simulink model "torqueBalancingJointControl"  (Simulink 8.0)
settings: Solver=FixedStepDiscrete  StartTime=0.0  StopTime=CONFIG.SIMULATION_TIME  FixedStep=CONFIG.Ts  RelTol=1e-3
InitFcn:
  | initTorqueBalancing;
undefined symbols (not defined in the file or in its folder): bVectorConstraints, CONFIG, ConstraintsMatrix, DiscIntNeverNeededParam, gain, reg, ROBOT_DOF, sat
libraries: WBToolboxLibrary x45, simulink x2
settings Model: Creator=daniele  LastModifiedBy=gnava
settings DebuggingCC: FcnCallInpInsideContextMsg=EnableAllAsWarning  FrameProcessingCompatibilityMsg=error
settings SFSimCC: SimParseCustomCode=off
settings CodeAppCC: CustomSymbolStrType=$N$R$M_T
settings GRTTargetCC: CodeReplacementLibrary=C89/C90 (ANSI)  CombineOutputUpdateFcns=off  GRTInterface=on

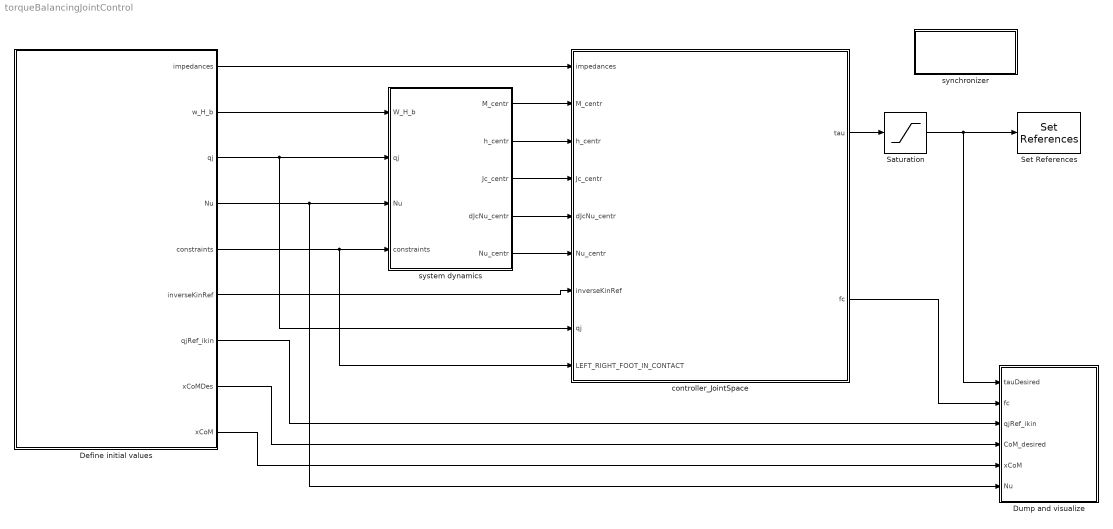
== system torqueBalancingJointControl ==
  Define initial values : Subsystem  Priority=-10
  Dump and visualize : Subsystem
  Saturation : Saturate  UpperLimit=sat.torque  LowerLimit=-sat.torque
  Set References : WBToolboxLibrary/wholeBodyActuators/Set References  controlType=Torque  robotName=WBT_robotName  localName=WBT_modelName  wbiFile=WBT_wbiFilename  wbiList=WBT_wbiList
  controller_JointSpace : Subsystem
  synchronizer : Subsystem
      mask Display: disp('SYNCHRONIZER')
  system dynamics : Subsystem
  wires:
  Define initial values/2(w_H_b) -> system dynamics/1(W_H_b)
  Define initial values/3(qj) -> system dynamics/2(qj), controller_JointSpace/8(qj)
  Define initial values/4(Nu) -> system dynamics/3(Nu), Dump and visualize/6(Nu)
  Define initial values/5(constraints) -> system dynamics/4(constraints), controller_JointSpace/9(LEFT_RIGHT_FOOT_IN_CONTACT)
  system dynamics/1(M_centr) -> controller_JointSpace/2(M_centr)
  system dynamics/2(h_centr) -> controller_JointSpace/3(h_centr)
  system dynamics/3(Jc_centr) -> controller_JointSpace/4(Jc_centr)
  system dynamics/4(dJcNu_centr) -> controller_JointSpace/5(dJcNu_centr)
  system dynamics/5(Nu_centr) -> controller_JointSpace/6(Nu_centr)
  Define initial values/6(inverseKinRef) -> controller_JointSpace/7(inverseKinRef)
  Define initial values/1(impedances) -> controller_JointSpace/1(impedances)
  controller_JointSpace/1("tau ") -> Saturation/1
  Saturation/1 -> Dump and visualize/1(tauDesired), Set References/1
  controller_JointSpace/2(fc) -> Dump and visualize/2(fc)
  Define initial values/7(qjRef_ikin) -> Dump and visualize/3(qjRef_ikin)
  Define initial values/8(xCoMDes) -> Dump and visualize/4(CoM_desired)
  Define initial values/9(xCoM) -> Dump and visualize/5(xCoM)

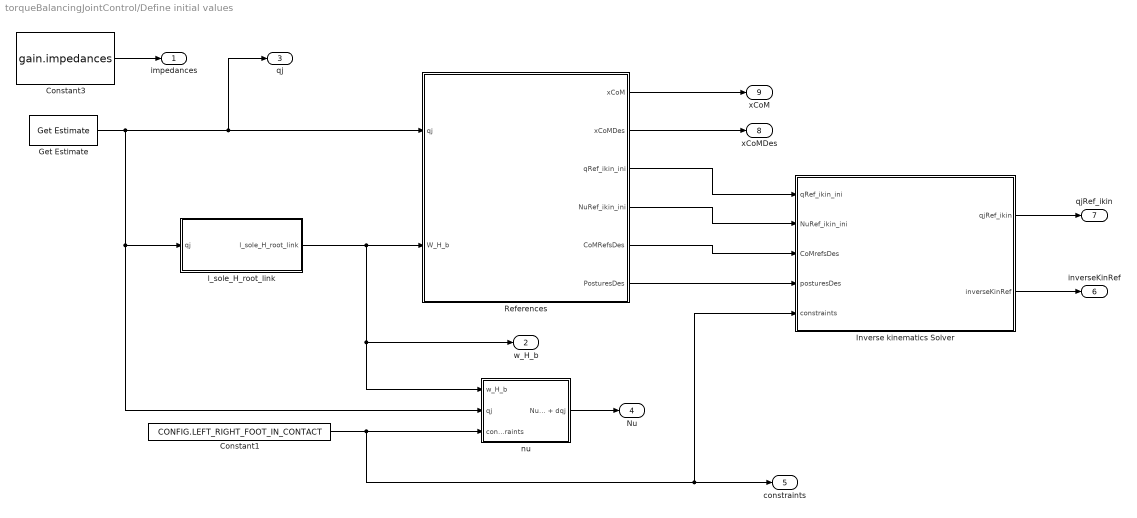
== system torqueBalancingJointControl/Define initial values ==
  Constant1 : Constant  Value=CONFIG.LEFT_RIGHT_FOOT_IN_CONTACT
  Constant3 : Constant  Value=gain.impedances
  Get Estimate : WBToolboxLibrary/wholeBodyStates/Get Estimate  estimateType=Joints Position  robotName=WBT_robotName  localName=WBT_modelName  wbiFile=WBT_wbiFilename  wbiList=WBT_wbiList
  Inverse kinematics Solver : Subsystem
  References : Subsystem
  l_sole_H_root_link : Subsystem
  nu : Subsystem
  impedances : Outport
  w_H_b : Outport  Port=2
  qj : Outport  Port=3
  Nu : Outport  Port=4
  constraints : Outport  Port=5
  inverseKinRef : Outport  Port=6
  qjRef_ikin : Outport  Port=7
  xCoMDes : Outport  Port=8
  xCoM : Outport  Port=9
  wires:
  Constant3/1 -> impedances/1
  Get Estimate/1 -> l_sole_H_root_link/1(qj), nu/2(qj), References/1(qj), qj/1
  l_sole_H_root_link/1(l_sole_H_root_link) -> w_H_b/1, nu/1(w_H_b), References/2(W_H_b)
  nu/1(Nu_b + dqj) -> Nu/1
  References/1(xCoM) -> xCoM/1
  References/2(xCoMDes) -> xCoMDes/1
  Constant1/1 -> Inverse kinematics Solver/5(constraints), constraints/1, nu/3("constraints ")
  Inverse kinematics Solver/1(qjRef_ikin) -> qjRef_ikin/1
  Inverse kinematics Solver/2(inverseKinRef) -> inverseKinRef/1
  References/6(PosturesDes) -> Inverse kinematics Solver/4(posturesDes)
  References/5(CoMRefsDes) -> Inverse kinematics Solver/3(CoMrefsDes)
  References/4(NuRef_ikin_ini) -> Inverse kinematics Solver/2(NuRef_ikin_ini)
  References/3(qRef_ikin_ini) -> Inverse kinematics Solver/1(qRef_ikin_ini)

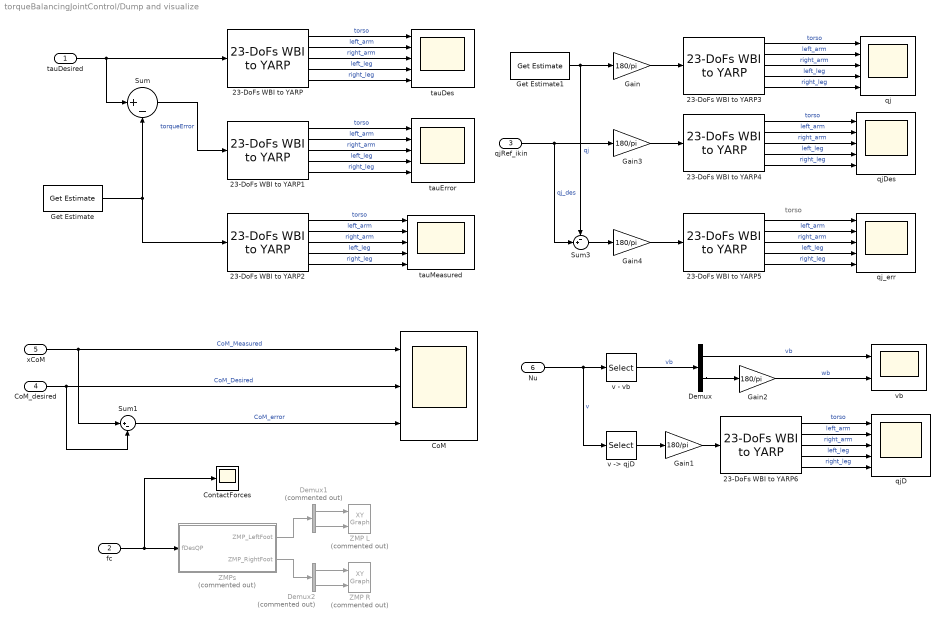
== system torqueBalancingJointControl/Dump and visualize ==
  note: torso
  tauDesired : Inport
  fc : Inport  Port=2
  qjRef_ikin : Inport  Port=3
  CoM_desired : Inport  Port=4
  xCoM : Inport  Port=5
  Nu : Inport  Port=6
  23-DoFs WBI to YARP{,1..6} (7 alike) : WBToolboxLibrary/Utilities/23-DoFs WBI to YARP
  CoM : Scope  NumInputPorts=3
      settings: ShowLegends=on  TimeRange=400  YMin=-0.2~-0.2~-0.045  YMax=0.6~0.6~0.005  SaveName=CoM_data
  ContactForces : Scope
      settings: SaveName=ScopeData2
  Demux : Demux  Outputs=2
  Demux1 : Demux  Commented=on  Outputs=2
  Demux2 : Demux  Commented=on  Outputs=2
  Gain{,1..4} (5 alike) : Gain  Gain=180/pi
  Get Estimate : WBToolboxLibrary/wholeBodyStates/Get Estimate  estimateType=Joints Torque  robotName=WBT_robotName  localName=WBT_modelName  wbiFile=WBT_wbiFilename  wbiList=WBT_wbiList
  Get Estimate1 : WBToolboxLibrary/wholeBodyStates/Get Estimate  estimateType=Joints Position  robotName=WBT_robotName  localName=WBT_modelName  wbiFile=WBT_wbiFilename  wbiList=WBT_wbiList
  Sum : Sum  Inputs=|+-
  Sum1 : Sum  Inputs=|+-
  Sum3 : Sum  Inputs=-+|
  ZMP L : simulink/Sinks/XY Graph  Commented=on  xmin=gain.footSize(1,1)  xmax=gain.footSize(1,2)  ymin=gain.footSize(2,1)  ymax=gain.footSize(2,2)  st=-1
  ZMP R : simulink/Sinks/XY Graph  Commented=on  xmin=gain.footSize(1,1)  xmax=gain.footSize(1,2)  ymin=gain.footSize(2,1)  ymax=gain.footSize(2,2)  st=-1
  ZMPs : Subsystem  Commented=on
  qj : Scope  NumInputPorts=5
      settings: ShowLegends=on  TimeRange=40  YMin=-5~-40~-40~-15~-15  YMax=8~60~60~15~15  SaveName=qj_and_v
  qjD : Scope  NumInputPorts=5
      settings: ShowLegends=on  TimeRange=40  YMin=-1~-0.2~-0.6~-3~-3  YMax=3~0.5~0.3~3~3  SaveName=qj_and_v1
  qjDes : Scope  NumInputPorts=5
      settings: ShowLegends=on  TimeRange=40  YMin=-13.18879~-50.35129~-51.01363~-14.07847~-15.42592  YMax=8.56867~62.73253~62.72359~15.05436~15.88206  SaveName=qj_and_v3
  qj_err : Scope  NumInputPorts=5
      settings: ShowLegends=on  TimeRange=40  YMin=-27.27476~-4.23851~-4.57478~-6.37088~-5.38345  YMax=17.10367~4.06727~2.87419~5.35549~6.40509  SaveName=qj_and_v4
  tauDes : Scope  NumInputPorts=5
      settings: ShowLegends=on  TimeRange=14  YMin=-19.49982~-5.04916~-6.41013~-19.61704~-14.11485  YMax=15.70467~4.10511~5.2534~18.2484~18.38621  SaveName=tauDes
  tauError : Scope  NumInputPorts=5
      settings: ShowLegends=on  TimeRange=90  YMin=-4.41555~-1.22651~-0.86191~-3.55477~-4.30808  YMax=5.88399~0.83922~1.20608~5.47683~6.35708  SaveName=tauError
  tauMeasured : Scope  NumInputPorts=5
      settings: ShowLegends=on  TimeRange=14  YMin=-6~-2.5~-2.5~-6~-6  YMax=5~2~1.5~5~5  SaveName=tauMeasured
  v - vb : Selector  InputPortWidth=ROBOT_DOF+6  IndexOptions=Index vector (dialog)  Indices=[1:6]  OutputSizes=1
  "v -> qjD" : Selector  InputPortWidth=ROBOT_DOF+6  IndexOptions=Index vector (dialog)  Indices=[7:ROBOT_DOF+6]  OutputSizes=1
  vb : Scope  NumInputPorts=2
      settings: ShowLegends=on  TimeRange=40  YMin=-0.02~-1.75  YMax=0.0175~2  SaveName=qj_and_v2
  wires:
  xCoM/1 -> Sum1/1, CoM/1  "CoM_Measured"
  CoM_desired/1 -> Sum1/2, CoM/2  "CoM_Desired"
  Nu/1 -> "v -> qjD"/1, v - vb/1  "v"
  Get Estimate1/1 -> Sum3/1, Gain/1  "qj"
  Gain/1 -> 23-DoFs WBI to YARP3/1
  23-DoFs WBI to YARP3/5 -> qj/5  "right_leg"
  23-DoFs WBI to YARP3/1 -> qj/1  "torso"
  23-DoFs WBI to YARP3/2 -> qj/2  "left_arm"
  23-DoFs WBI to YARP3/4 -> qj/4  "left_leg"
  23-DoFs WBI to YARP3/3 -> qj/3  "right_arm"
  23-DoFs WBI to YARP6/5 -> qjD/5  "right_leg"
  23-DoFs WBI to YARP6/1 -> qjD/1  "torso"
  23-DoFs WBI to YARP6/2 -> qjD/2  "left_arm"
  23-DoFs WBI to YARP6/4 -> qjD/4  "left_leg"
  23-DoFs WBI to YARP6/3 -> qjD/3  "right_arm"
  "v -> qjD"/1 -> Gain1/1
  v - vb/1 -> Demux/1  "vb"
  Demux/1 -> vb/1  "vb"
  Demux/2 -> Gain2/1
  Gain1/1 -> 23-DoFs WBI to YARP6/1
  Gain2/1 -> vb/2  "wb"
  fc/1 -> ContactForces/1, ZMPs/1(fDesQP)
  ZMPs/1(ZMP_LeftFoot) -> Demux1/1
  ZMPs/2(ZMP_RightFoot) -> Demux2/1
  Demux1/1 -> ZMP L/1
  Demux1/2 -> ZMP L/2
  Demux2/1 -> ZMP R/1
  Demux2/2 -> ZMP R/2
  tauDesired/1 -> Sum/1, 23-DoFs WBI to YARP/1
  Get Estimate/1 -> 23-DoFs WBI to YARP2/1, Sum/2
  23-DoFs WBI to YARP/5 -> tauDes/5  "right_leg"
  23-DoFs WBI to YARP/1 -> tauDes/1  "torso"
  23-DoFs WBI to YARP/2 -> tauDes/2  "left_arm"
  23-DoFs WBI to YARP/4 -> tauDes/4  "left_leg"
  23-DoFs WBI to YARP/3 -> tauDes/3  "right_arm"
  23-DoFs WBI to YARP1/5 -> tauError/5  "right_leg"
  23-DoFs WBI to YARP1/1 -> tauError/1  "torso"
  23-DoFs WBI to YARP1/2 -> tauError/2  "left_arm"
  23-DoFs WBI to YARP1/4 -> tauError/4  "left_leg"
  23-DoFs WBI to YARP1/3 -> tauError/3  "right_arm"
  Sum/1 -> 23-DoFs WBI to YARP1/1  "torqueError"
  23-DoFs WBI to YARP2/5 -> tauMeasured/5  "right_leg"
  23-DoFs WBI to YARP2/1 -> tauMeasured/1  "torso"
  23-DoFs WBI to YARP2/2 -> tauMeasured/2  "left_arm"
  23-DoFs WBI to YARP2/4 -> tauMeasured/4  "left_leg"
  23-DoFs WBI to YARP2/3 -> tauMeasured/3  "right_arm"
  23-DoFs WBI to YARP4/5 -> qjDes/5  "right_leg"
  23-DoFs WBI to YARP4/1 -> qjDes/1  "torso"
  23-DoFs WBI to YARP4/2 -> qjDes/2  "left_arm"
  23-DoFs WBI to YARP4/4 -> qjDes/4  "left_leg"
  23-DoFs WBI to YARP4/3 -> qjDes/3  "right_arm"
  Gain4/1 -> 23-DoFs WBI to YARP5/1
  23-DoFs WBI to YARP5/5 -> qj_err/5  "right_leg"
  23-DoFs WBI to YARP5/2 -> qj_err/2  "left_arm"
  23-DoFs WBI to YARP5/4 -> qj_err/4  "left_leg"
  23-DoFs WBI to YARP5/3 -> qj_err/3  "right_arm"
  Sum3/1 -> Gain4/1
  qjRef_ikin/1 -> Gain3/1, Sum3/2  "qj_des"
  Gain3/1 -> 23-DoFs WBI to YARP4/1
  23-DoFs WBI to YARP5/1 -> qj_err/1
  Sum1/1 -> CoM/3  "CoM_error"

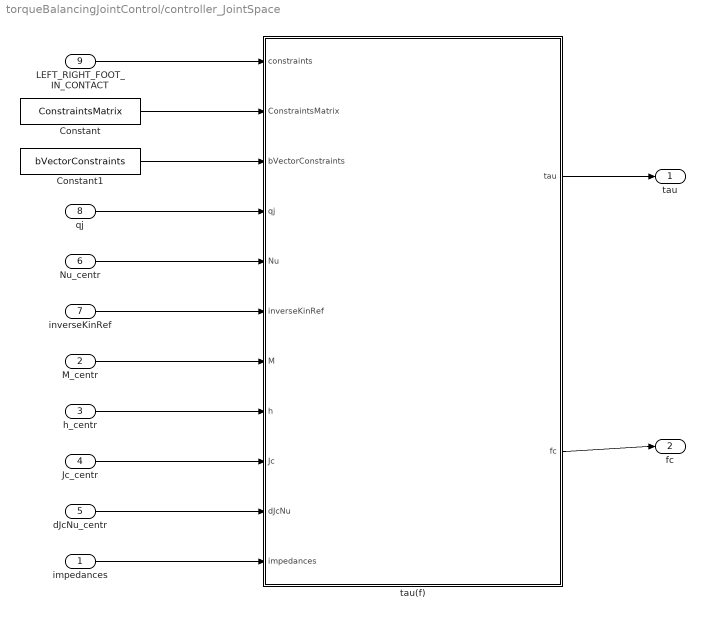
== system torqueBalancingJointControl/controller_JointSpace ==
  impedances : Inport
  M_centr : Inport  Port=2
  h_centr : Inport  Port=3
  Jc_centr : Inport  Port=4
  dJcNu_centr : Inport  Port=5
  Nu_centr : Inport  Port=6
  inverseKinRef : Inport  Port=7
  qj : Inport  Port=8
  LEFT_RIGHT_FOOT_IN_CONTACT : Inport  Port=9
  Constant : Constant  Value=ConstraintsMatrix
  Constant1 : Constant  Value=bVectorConstraints
  "tau(f) " : MATLAB Function  TreatAsAtomicUnit=on
  "tau " : Outport
  fc : Outport  Port=2
  wires:
  LEFT_RIGHT_FOOT_IN_CONTACT/1 -> "tau(f) "/1(constraints)
  M_centr/1 -> "tau(f) "/7(M)
  h_centr/1 -> "tau(f) "/8(h)
  Constant/1 -> "tau(f) "/2(ConstraintsMatrix)
  Constant1/1 -> "tau(f) "/3(bVectorConstraints)
  Jc_centr/1 -> "tau(f) "/9(Jc)
  dJcNu_centr/1 -> "tau(f) "/10(dJcNu)
  Nu_centr/1 -> "tau(f) "/5(Nu)
  impedances/1 -> "tau(f) "/11(impedances)
  "tau(f) "/1(tau) -> "tau "/1
  qj/1 -> "tau(f) "/4(qj)
  inverseKinRef/1 -> "tau(f) "/6(inverseKinRef)
  "tau(f) "/2(fc) -> fc/1

== system torqueBalancingJointControl/synchronizer ==
  Real Time Synchronizer : WBToolboxLibrary/Utilities/Real Time Synchronizer  Commented=on  period=CONFIG.Ts
  Simulator Synchronizer : WBToolboxLibrary/Utilities/Simulator Synchronizer  period=CONFIG.Ts  serverPortName='/clock/rpc'  clientPortName='/WBT_synchronizer/rpc:o'

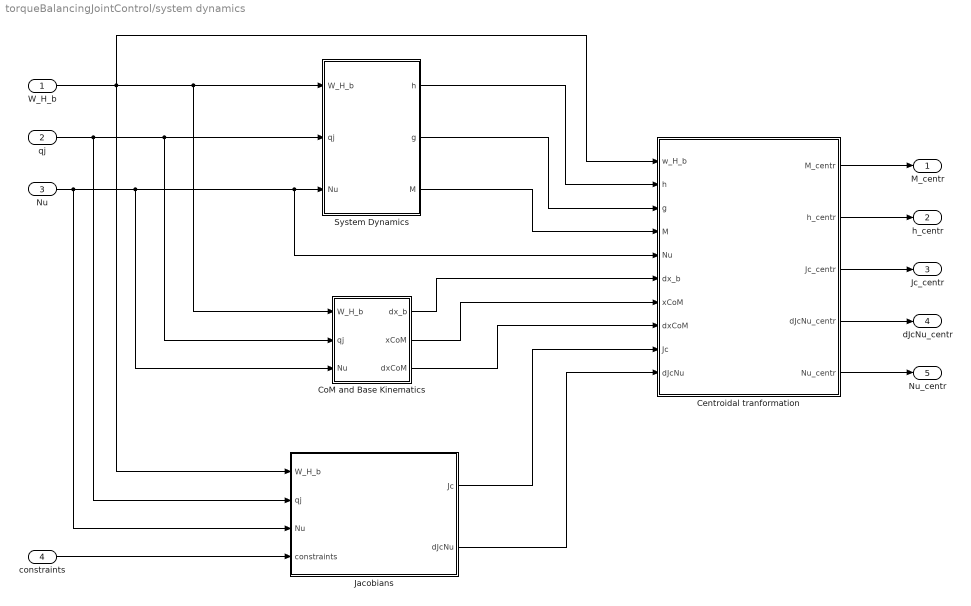
== system torqueBalancingJointControl/system dynamics ==
  W_H_b : Inport
  qj : Inport  Port=2
  Nu : Inport  Port=3
  constraints : Inport  Port=4
  Centroidal tranformation : Subsystem
  CoM and Base Kinematics : Subsystem
  Jacobians : Subsystem
  System Dynamics : Subsystem
  M_centr : Outport
  h_centr : Outport  Port=2
  Jc_centr : Outport  Port=3
  dJcNu_centr : Outport  Port=4
  Nu_centr : Outport  Port=5
  wires:
  Jacobians/2(dJcNu) -> Centroidal tranformation/10(dJcNu)
  Centroidal tranformation/1(M_centr) -> M_centr/1
  System Dynamics/1(h) -> Centroidal tranformation/2(h)
  System Dynamics/2(g) -> Centroidal tranformation/3(g)
  System Dynamics/3(M) -> Centroidal tranformation/4(M)
  CoM and Base Kinematics/1(dx_b) -> Centroidal tranformation/6(dx_b)
  CoM and Base Kinematics/2(xCoM) -> Centroidal tranformation/7(xCoM)
  CoM and Base Kinematics/3(dxCoM) -> Centroidal tranformation/8(dxCoM)
  Jacobians/1(Jc) -> Centroidal tranformation/9(Jc)
  qj/1 -> Jacobians/2(qj), CoM and Base Kinematics/2(qj), System Dynamics/2(qj)
  Nu/1 -> Jacobians/3(Nu), CoM and Base Kinematics/3(Nu), Centroidal tranformation/5(Nu), System Dynamics/3(Nu)
  W_H_b/1 -> Centroidal tranformation/1(w_H_b), Jacobians/1(W_H_b), System Dynamics/1(W_H_b), CoM and Base Kinematics/1(W_H_b)
  Centroidal tranformation/3(Jc_centr) -> Jc_centr/1
  Centroidal tranformation/2(h_centr) -> h_centr/1
  constraints/1 -> Jacobians/4(constraints)
  Centroidal tranformation/5(Nu_centr) -> Nu_centr/1
  Centroidal tranformation/4(dJcNu_centr) -> dJcNu_centr/1

== system torqueBalancingJointControl/Define initial values/Inverse kinematics Solver ==
  qRef_ikin_ini : Inport
  NuRef_ikin_ini : Inport  Port=2
  CoMrefsDes : Inport  Port=3
  posturesDes : Inport  Port=4
  constraints : Inport  Port=5
  Generate ikin Errors : Subsystem
  ikin visualizer : Subsystem
  ikin_DoubleIntegrator : Subsystem
  ikin_utilities : Subsystem
  trajectoryGeneratorCoM : MATLAB Function  TreatAsAtomicUnit=on
  qjRef_ikin : Outport
  inverseKinRef : Outport  Port=2
  wires:
  Generate ikin Errors/1(iKinFeetCorr) -> trajectoryGeneratorCoM/1(iKinFeetCorr), ikin visualizer/1(Ikin_feetCorr)
  Generate ikin Errors/2(iKinComCorr) -> trajectoryGeneratorCoM/2(iKinComCorr), ikin visualizer/2(Ikin_CoMCorr)
  Generate ikin Errors/3(iKinPostCorr) -> ikin visualizer/3(Ikin_PostCorr), trajectoryGeneratorCoM/3(iKinPostCorr)
  ikin_DoubleIntegrator/2(qRef_ikin) -> ikin_utilities/1(qRef_ikin), Generate ikin Errors/12(qRef_ikin)
  ikin_DoubleIntegrator/1(NuRef_ikin) -> ikin_utilities/2(NuRef_ikin), Generate ikin Errors/11(NuRef_iKin)
  qRef_ikin_ini/1 -> ikin_DoubleIntegrator/3(qRef_ikin_init), ikin_utilities/3(qRef_ikin_init)
  CoMrefsDes/1 -> Generate ikin Errors/1(CoMrefsDes)
  posturesDes/1 -> Generate ikin Errors/2(posturesDes)
  ikin_utilities/1(Jlsole) -> Generate ikin Errors/3(Jlfoot), trajectoryGeneratorCoM/4(J_lfoot)
  ikin_utilities/2(Jrsole) -> trajectoryGeneratorCoM/5(J_rfoot), Generate ikin Errors/4(Jrfoot)
  ikin_utilities/3(JCoM) -> Generate ikin Errors/5(JCoM), trajectoryGeneratorCoM/6(J_com)
  ikin_utilities/4(deltaRFootPos) -> Generate ikin Errors/6(rfootPos)
  ikin_utilities/5(deltaLFootPos) -> Generate ikin Errors/7(lfootPos)
  ikin_utilities/6(CoMPos) -> Generate ikin Errors/8(CoMPos)
  ikin_utilities/7(deltaLFootOri) -> Generate ikin Errors/9(lfootOri)
  ikin_utilities/8(deltaRFootOri) -> Generate ikin Errors/10(rfootOri)
  NuRef_ikin_ini/1 -> ikin_DoubleIntegrator/2(Nu_ikin_init)
  trajectoryGeneratorCoM/1(dNuRef_ikin) -> ikin_DoubleIntegrator/1(dNuRef_ikin)
  constraints/1 -> trajectoryGeneratorCoM/10(constraints)
  ikin_utilities/9(dJlfootNu) -> trajectoryGeneratorCoM/7(dJcNu_lf)
  ikin_utilities/10(dJrfootNu) -> trajectoryGeneratorCoM/8(dJcNu_rf)
  ikin_utilities/11(dJCoMNu) -> trajectoryGeneratorCoM/9(dJ_comNu)
  ikin_DoubleIntegrator/3(inverseKinRef) -> inverseKinRef/1
  ikin_DoubleIntegrator/4(qjRef_ikin) -> qjRef_ikin/1

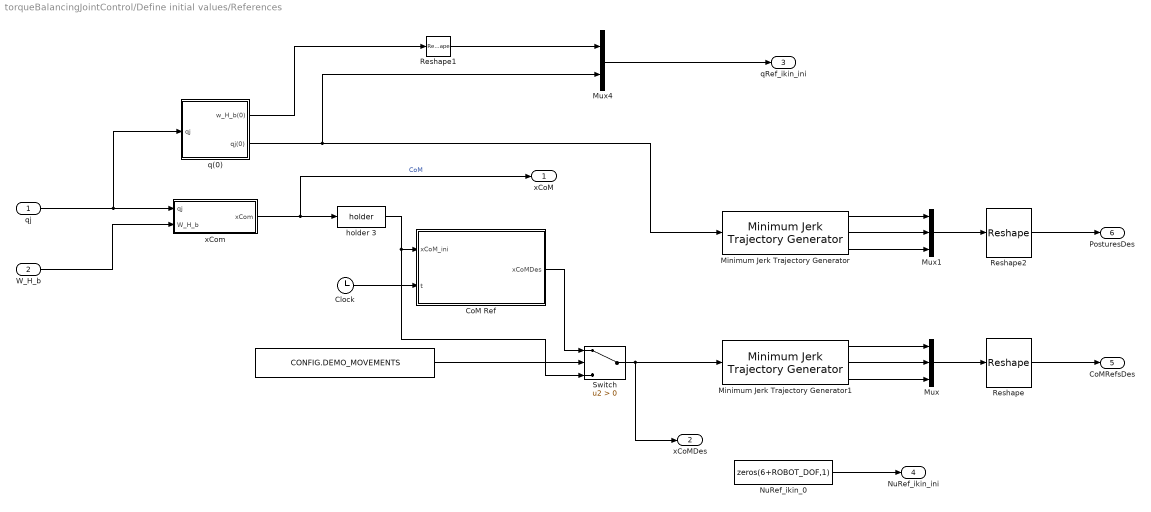
== system torqueBalancingJointControl/Define initial values/References ==
  qj : Inport
  W_H_b : Inport  Port=2
  " " : Constant  Value=CONFIG.DEMO_MOVEMENTS
  Clock : Clock
  CoM Ref : MATLAB Function  TreatAsAtomicUnit=on
  Minimum Jerk Trajectory Generator : WBToolboxLibrary/Utilities/Minimum Jerk Trajectory Generator  externalSettlingTime=off  settlingTime=3  sampleTime=CONFIG.Ts  firstDerivatives=on  secondDerivatives=on  explicitInitialValue=off
  Minimum Jerk Trajectory Generator1 : WBToolboxLibrary/Utilities/Minimum Jerk Trajectory Generator  externalSettlingTime=off  settlingTime=3  sampleTime=CONFIG.Ts  firstDerivatives=on  secondDerivatives=on  explicitInitialValue=off
  Mux : Mux  Inputs=3
  Mux1 : Mux  Inputs=3
  Mux4 : Mux  Inputs=2
  NuRef_ikin_0 : Constant  Value=zeros(6+ROBOT_DOF,1)
  Reshape : Reshape  OutputDimensionality=Customize  OutputDimensions=[3,3]
  Reshape1 : Reshape
  Reshape2 : Reshape  OutputDimensionality=Customize  OutputDimensions=[ROBOT_DOF,3]
  Switch : Switch  Criteria=u2 > Threshold
  holder 3 : WBToolboxLibrary/Utilities/holder 
  q(0) : Subsystem
  xCom : Subsystem  Priority=-2
  xCoM : Outport
  xCoMDes : Outport  Port=2
  qRef_ikin_ini : Outport  Port=3
  NuRef_ikin_ini : Outport  Port=4
  CoMRefsDes : Outport  Port=5
  PosturesDes : Outport  Port=6
  wires:
  xCom/1(xCom) -> xCoM/1, holder 3/1  "CoM"
  qj/1 -> xCom/1(qj), q(0)/1(qj)
  Reshape1/1 -> Mux4/1
  q(0)/1(w_H_b(0)) -> Reshape1/1
  q(0)/2(qj(0)) -> Minimum Jerk Trajectory Generator/1, Mux4/2
  Mux4/1 -> qRef_ikin_ini/1
  Minimum Jerk Trajectory Generator1/1 -> Mux/1
  Minimum Jerk Trajectory Generator1/2 -> Mux/2
  Minimum Jerk Trajectory Generator1/3 -> Mux/3
  Mux/1 -> Reshape/1
  Minimum Jerk Trajectory Generator/1 -> Mux1/1
  Minimum Jerk Trajectory Generator/2 -> Mux1/2
  Minimum Jerk Trajectory Generator/3 -> Mux1/3
  Mux1/1 -> Reshape2/1
  NuRef_ikin_0/1 -> NuRef_ikin_ini/1
  Reshape2/1 -> PosturesDes/1
  Reshape/1 -> CoMRefsDes/1
  W_H_b/1 -> xCom/2(W_H_b)
  " "/1 -> Switch/2
  holder 3/1 -> Switch/3, CoM Ref/1(xCoM_ini)
  Switch/1 -> xCoMDes/1, Minimum Jerk Trajectory Generator1/1
  Clock/1 -> CoM Ref/2(t)
  CoM Ref/1(xCoMDes) -> Switch/1

== system torqueBalancingJointControl/Define initial values/l_sole_H_root_link ==
  qj : Inport
  Constant5 : Constant  Value=eye(4)
  Constant6 : Constant  Value=eye(4)
  Inv\* : Product  Inputs=/*  Multiplication=Matrix(*)
  l_sole : WBToolboxLibrary/wholeBodyModel/Kinematics/Forward Kinematics  frameName='l_sole'  robotName=WBT_robotName  localName=WBT_modelName  wbiFile=WBT_wbiFilename  wbiList=WBT_wbiList
  root_link : WBToolboxLibrary/wholeBodyModel/Kinematics/Forward Kinematics  frameName='root_link'  robotName=WBT_robotName  localName=WBT_modelName  wbiFile=WBT_wbiFilename  wbiList=WBT_wbiList
  l_sole_H_root_link : Outport
  wires:
  Constant5/1 -> l_sole/1
  Inv\*/1 -> l_sole_H_root_link/1  "l_sole_H_root_link"
  l_sole/1 -> Inv\*/1
  Constant6/1 -> root_link/1
  qj/1 -> root_link/2, l_sole/2
  root_link/1 -> Inv\*/2

== system torqueBalancingJointControl/Define initial values/nu ==
  w_H_b : Inport
  qj : Inport  Port=2
  "constraints " : Inport  Port=3
  Get Estimate : WBToolboxLibrary/wholeBodyStates/Get Estimate  estimateType=Joints Velocity  robotName=WBT_robotName  localName=WBT_modelName  wbiFile=WBT_wbiFilename  wbiList=WBT_wbiList
  Jacobian l_sole : WBToolboxLibrary/wholeBodyModel/Jacobians/Jacobian  frameName='l_sole'  robotName=WBT_robotName  localName=WBT_modelName  wbiFile=WBT_wbiFilename  wbiList=WBT_wbiList
  Jacobian r_sole : WBToolboxLibrary/wholeBodyModel/Jacobians/Jacobian  frameName='r_sole'  robotName=WBT_robotName  localName=WBT_modelName  wbiFile=WBT_wbiFilename  wbiList=WBT_wbiList
  Mux : Mux  Inputs=2
  genBaseVelocity : MATLAB Function  TreatAsAtomicUnit=on
  Nu_b + dqj : Outport
  wires:
  Get Estimate/1 -> genBaseVelocity/4(dq), Mux/2
  Mux/1 -> Nu_b + dqj/1
  Jacobian r_sole/1 -> genBaseVelocity/2(JcRightFoot)
  "constraints "/1 -> genBaseVelocity/3(Constraints)
  genBaseVelocity/1(Nu_base) -> Mux/1
  Jacobian l_sole/1 -> genBaseVelocity/1(JcLeftFoot)
  qj/1 -> Jacobian l_sole/2, Jacobian r_sole/2
  w_H_b/1 -> Jacobian r_sole/1, Jacobian l_sole/1

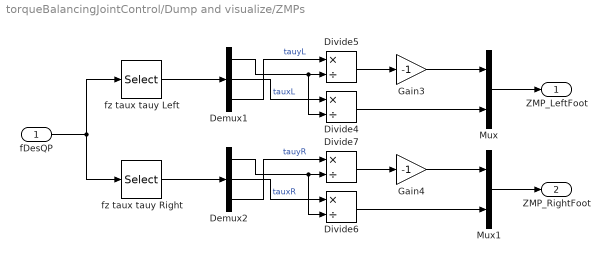
== system torqueBalancingJointControl/Dump and visualize/ZMPs ==
  fDesQP : Inport
  Demux1 : Demux  Outputs=3
  Demux2 : Demux  Outputs=3
  Divide{4..7} (4 alike) : Product  Inputs=*/
  Gain3 : Gain  Gain=-1
  Gain4 : Gain  Gain=-1
  Mux : Mux  Inputs=2
  Mux1 : Mux  Inputs=2
  fz taux tauy Left : Selector  InputPortWidth=12  IndexOptions=Index vector (dialog)  Indices=[3 4 5]  OutputSizes=1
  fz taux tauy Right : Selector  InputPortWidth=12  IndexOptions=Index vector (dialog)  Indices=[9 10 11]  OutputSizes=1
  ZMP_LeftFoot : Outport
  ZMP_RightFoot : Outport  Port=2
  wires:
  fz taux tauy Left/1 -> Demux1/1
  Demux1/1 -> Divide4/2, Divide5/2
  Divide7/1 -> Gain4/1
  Divide4/1 -> Mux/2
  Divide5/1 -> Gain3/1
  fz taux tauy Right/1 -> Demux2/1
  Demux2/1 -> Divide6/2, Divide7/2
  fDesQP/1 -> fz taux tauy Left/1, fz taux tauy Right/1
  Gain3/1 -> Mux/1
  Mux/1 -> ZMP_LeftFoot/1
  Divide6/1 -> Mux1/2
  Gain4/1 -> Mux1/1
  Mux1/1 -> ZMP_RightFoot/1
  Demux1/2 -> Divide4/1  "tauxL"
  Demux1/3 -> Divide5/1  "tauyL"
  Demux2/2 -> Divide6/1  "tauxR"
  Demux2/3 -> Divide7/1  "tauyR"

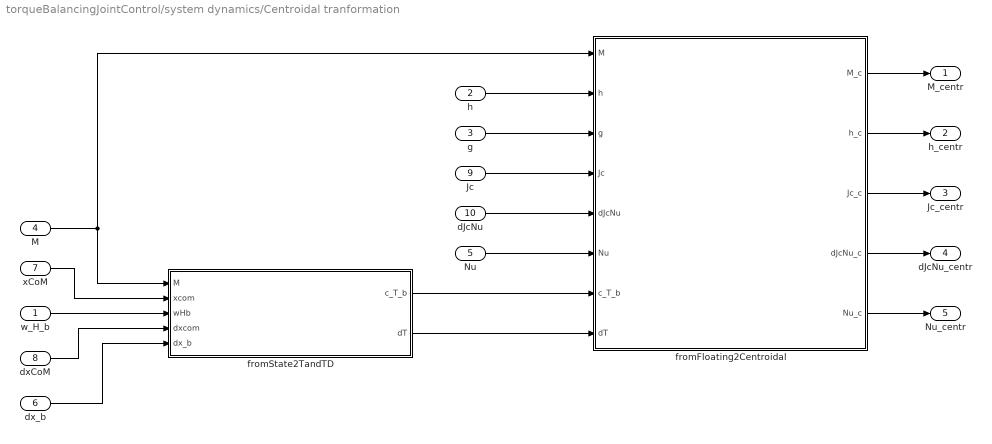
== system torqueBalancingJointControl/system dynamics/Centroidal tranformation ==
  w_H_b : Inport
  h : Inport  Port=2
  g : Inport  Port=3
  M : Inport  Port=4
  Nu : Inport  Port=5
  dx_b : Inport  Port=6
  xCoM : Inport  Port=7
  dxCoM : Inport  Port=8
  Jc : Inport  Port=9
  dJcNu : Inport  Port=10
  fromFloating2Centroidal : MATLAB Function  TreatAsAtomicUnit=on
  fromState2TandTD : MATLAB Function  TreatAsAtomicUnit=on
  M_centr : Outport
  h_centr : Outport  Port=2
  Jc_centr : Outport  Port=3
  dJcNu_centr : Outport  Port=4
  Nu_centr : Outport  Port=5
  wires:
  Nu/1 -> fromFloating2Centroidal/6(Nu)
  dx_b/1 -> fromState2TandTD/5(dx_b)
  xCoM/1 -> fromState2TandTD/2(xcom)
  fromState2TandTD/2(dT) -> fromFloating2Centroidal/8(dT)
  h/1 -> fromFloating2Centroidal/2(h)
  g/1 -> fromFloating2Centroidal/3(g)
  dxCoM/1 -> fromState2TandTD/4(dxcom)
  w_H_b/1 -> fromState2TandTD/3(wHb)
  fromState2TandTD/1(c_T_b) -> fromFloating2Centroidal/7(c_T_b)
  dJcNu/1 -> fromFloating2Centroidal/5(dJcNu)
  Jc/1 -> fromFloating2Centroidal/4(Jc)
  M/1 -> fromState2TandTD/1(M), fromFloating2Centroidal/1(M)
  fromFloating2Centroidal/1(M_c) -> M_centr/1
  fromFloating2Centroidal/2(h_c) -> h_centr/1
  fromFloating2Centroidal/3(Jc_c) -> Jc_centr/1
  fromFloating2Centroidal/4(dJcNu_c) -> dJcNu_centr/1
  fromFloating2Centroidal/5(Nu_c) -> Nu_centr/1

== system torqueBalancingJointControl/system dynamics/CoM and Base Kinematics ==
  W_H_b : Inport
  qj : Inport  Port=2
  Nu : Inport  Port=3
  "CoM6D ->  CoMXYZ1" : Selector  InputPortWidth=6  IndexOptions=Index vector (dialog)  Indices=[1 2 3]  OutputSizes=1
  "CoM6D ->  CoMXYZ4" : Selector  InputPortWidth=6+ROBOT_DOF  IndexOptions=Index vector (dialog)  Indices=[1 2 3]  OutputSizes=1
  "CoM6D ->  CoMXYZ5" : Selector  NumberOfDimensions=2  InputPortWidth=7  IndexOptions=Index vector (dialog),Index vector (dialog)  Indices=[1 2 3],[4]  OutputSizes=1,1
  Jacobian CoM : WBToolboxLibrary/wholeBodyModel/Jacobians/Jacobian  frameName='com'  robotName=WBT_robotName  localName=WBT_modelName  wbiFile=WBT_wbiFilename  wbiList=WBT_wbiList
  JcNu : Product  Multiplication=Matrix(*)
  com : WBToolboxLibrary/wholeBodyModel/Kinematics/Forward Kinematics  frameName='com'  robotName=WBT_robotName  localName=WBT_modelName  wbiFile=WBT_wbiFilename  wbiList=WBT_wbiList
  dx_b : Outport
  xCoM : Outport  Port=2
  dxCoM : Outport  Port=3
  wires:
  qj/1 -> Jacobian CoM/2, com/2
  "CoM6D ->  CoMXYZ4"/1 -> dx_b/1
  com/1 -> "CoM6D ->  CoMXYZ5"/1
  "CoM6D ->  CoMXYZ5"/1 -> xCoM/1
  Jacobian CoM/1 -> JcNu/1
  Nu/1 -> JcNu/2, "CoM6D ->  CoMXYZ4"/1
  W_H_b/1 -> Jacobian CoM/1, com/1
  JcNu/1 -> "CoM6D ->  CoMXYZ1"/1
  "CoM6D ->  CoMXYZ1"/1 -> dxCoM/1

== system torqueBalancingJointControl/system dynamics/Jacobians ==
  W_H_b : Inport
  qj : Inport  Port=2
  Nu : Inport  Port=3
  constraints : Inport  Port=4
  "CoM6D ->  CoMXYZ3" : Selector  InputPortWidth=6+ROBOT_DOF  IndexOptions=Index vector (dialog)  Indices=[7:6+ROBOT_DOF]  OutputSizes=1
  "CoM6D ->  CoMXYZ4" : Selector  InputPortWidth=6+ROBOT_DOF  IndexOptions=Index vector (dialog)  Indices=[1 2 3 4 5 6]  OutputSizes=1
  DotJ Nu lFoot : WBToolboxLibrary/wholeBodyModel/Jacobians/DotJ Nu  frameName='l_sole'  robotName=WBT_robotName  localName=WBT_modelName  wbiFile=WBT_wbiFilename  wbiList=WBT_wbiList
  DotJ Nu rFoot : WBToolboxLibrary/wholeBodyModel/Jacobians/DotJ Nu  frameName='r_sole'  robotName=WBT_robotName  localName=WBT_modelName  wbiFile=WBT_wbiFilename  wbiList=WBT_wbiList
  Jacobian lFoot : WBToolboxLibrary/wholeBodyModel/Jacobians/Jacobian  frameName='l_sole'  robotName=WBT_robotName  localName=WBT_modelName  wbiFile=WBT_wbiFilename  wbiList=WBT_wbiList
  Jacobian rFoot : WBToolboxLibrary/wholeBodyModel/Jacobians/Jacobian  frameName='r_sole'  robotName=WBT_robotName  localName=WBT_modelName  wbiFile=WBT_wbiFilename  wbiList=WBT_wbiList
  composingSmoothJacobians : MATLAB Function  TreatAsAtomicUnit=on
  Jc : Outport
  dJcNu : Outport  Port=2
  wires:
  composingSmoothJacobians/1(Jc) -> Jc/1
  W_H_b/1 -> DotJ Nu rFoot/1, DotJ Nu lFoot/1, Jacobian rFoot/1, Jacobian lFoot/1
  qj/1 -> DotJ Nu rFoot/2, DotJ Nu lFoot/2, Jacobian rFoot/2, Jacobian lFoot/2
  constraints/1 -> composingSmoothJacobians/1(constraints)
  "CoM6D ->  CoMXYZ3"/1 -> DotJ Nu lFoot/4, DotJ Nu rFoot/4
  "CoM6D ->  CoMXYZ4"/1 -> DotJ Nu rFoot/3, DotJ Nu lFoot/3
  composingSmoothJacobians/2(dJcNu) -> dJcNu/1
  DotJ Nu rFoot/1 -> composingSmoothJacobians/5(dJRNu)
  Jacobian lFoot/1 -> composingSmoothJacobians/2(JL)
  Jacobian rFoot/1 -> composingSmoothJacobians/3(JR)
  DotJ Nu lFoot/1 -> composingSmoothJacobians/4(dJLNu)
  Nu/1 -> "CoM6D ->  CoMXYZ3"/1, "CoM6D ->  CoMXYZ4"/1

== system torqueBalancingJointControl/system dynamics/System Dynamics ==
  W_H_b : Inport
  qj : Inport  Port=2
  Nu : Inport  Port=3
  "CoM6D ->  CoMXYZ3" : Selector  InputPortWidth=6+ROBOT_DOF  IndexOptions=Index vector (dialog)  Indices=[7:6+ROBOT_DOF]  OutputSizes=1
  "CoM6D ->  CoMXYZ4" : Selector  InputPortWidth=6+ROBOT_DOF  IndexOptions=Index vector (dialog)  Indices=[1 2 3 4 5 6]  OutputSizes=1
  Get Bias Forces : WBToolboxLibrary/wholeBodyModel/Dynamics/Get Bias Forces  robotName=WBT_robotName  localName=WBT_modelName  wbiFile=WBT_wbiFilename  wbiList=WBT_wbiList  explicitGravity=off
  Get Gravity Forces : WBToolboxLibrary/wholeBodyModel/Dynamics/Get Gravity Forces  robotName=WBT_robotName  localName=WBT_modelName  wbiFile=WBT_wbiFilename  wbiList=WBT_wbiList  explicitGravity=off
  Mass Matrix : WBToolboxLibrary/wholeBodyModel/Dynamics/Mass Matrix  robotName=WBT_robotName  localName=WBT_modelName  wbiFile=WBT_wbiFilename  wbiList=WBT_wbiList
  h : Outport
  g : Outport  Port=2
  M : Outport  Port=3
  wires:
  Mass Matrix/1 -> M/1
  Nu/1 -> "CoM6D ->  CoMXYZ3"/1, "CoM6D ->  CoMXYZ4"/1
  W_H_b/1 -> Get Bias Forces/1, Get Gravity Forces/1, Mass Matrix/1
  qj/1 -> Get Bias Forces/2, Get Gravity Forces/2, Mass Matrix/2
  "CoM6D ->  CoMXYZ4"/1 -> Get Bias Forces/3
  "CoM6D ->  CoMXYZ3"/1 -> Get Bias Forces/4
  Get Bias Forces/1 -> h/1
  Get Gravity Forces/1 -> g/1

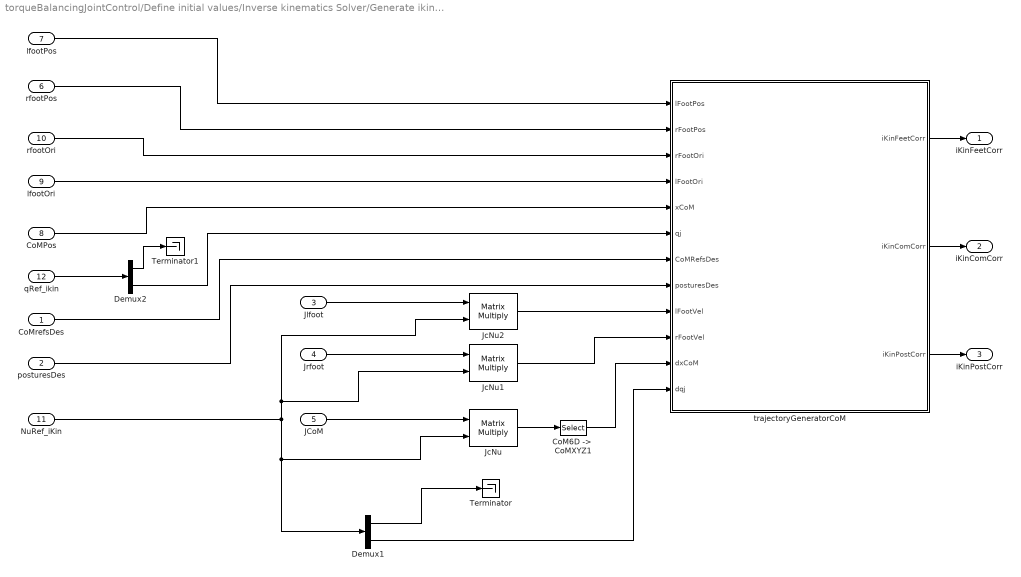
== system torqueBalancingJointControl/Define initial values/Inverse kinematics Solver/Generate ikin Errors ==
  CoMrefsDes : Inport
  posturesDes : Inport  Port=2
  Jlfoot : Inport  Port=3
  Jrfoot : Inport  Port=4
  JCoM : Inport  Port=5
  rfootPos : Inport  Port=6
  lfootPos : Inport  Port=7
  CoMPos : Inport  Port=8
  lfootOri : Inport  Port=9
  rfootOri : Inport  Port=10
  NuRef_iKin : Inport  Port=11
  qRef_ikin : Inport  Port=12
  "CoM6D ->  CoMXYZ1" : Selector  InputPortWidth=6  IndexOptions=Index vector (dialog)  Indices=[1 2 3]  OutputSizes=1
  Demux1 : Demux  Outputs=[6,ROBOT_DOF]
  Demux2 : Demux  Outputs=[16,ROBOT_DOF]
  JcNu : Product  Multiplication=Matrix(*)
  JcNu1 : Product  Multiplication=Matrix(*)
  JcNu2 : Product  Multiplication=Matrix(*)
  Terminator : Terminator
  Terminator1 : Terminator
  trajectoryGeneratorCoM : MATLAB Function  TreatAsAtomicUnit=on
  iKinFeetCorr : Outport
  iKinComCorr : Outport  Port=2
  iKinPostCorr : Outport  Port=3
  wires:
  Jrfoot/1 -> JcNu1/1
  trajectoryGeneratorCoM/1(iKinFeetCorr) -> iKinFeetCorr/1
  Demux1/1 -> Terminator/1
  CoMPos/1 -> trajectoryGeneratorCoM/5(xCoM)
  trajectoryGeneratorCoM/2(iKinComCorr) -> iKinComCorr/1
  Jlfoot/1 -> JcNu2/1
  CoMrefsDes/1 -> trajectoryGeneratorCoM/7(CoMRefsDes)
  JcNu/1 -> "CoM6D ->  CoMXYZ1"/1
  lfootPos/1 -> trajectoryGeneratorCoM/1(lFootPos)
  trajectoryGeneratorCoM/3(iKinPostCorr) -> iKinPostCorr/1
  JCoM/1 -> JcNu/1
  rfootPos/1 -> trajectoryGeneratorCoM/2(rFootPos)
  NuRef_iKin/1 -> Demux1/1, JcNu/2, JcNu2/2, JcNu1/2
  rfootOri/1 -> trajectoryGeneratorCoM/3(rFootOri)
  lfootOri/1 -> trajectoryGeneratorCoM/4(lFootOri)
  posturesDes/1 -> trajectoryGeneratorCoM/8(posturesDes)
  JcNu2/1 -> trajectoryGeneratorCoM/9(lFootVel)
  JcNu1/1 -> trajectoryGeneratorCoM/10(rFootVel)
  "CoM6D ->  CoMXYZ1"/1 -> trajectoryGeneratorCoM/11(dxCoM)
  Demux1/2 -> trajectoryGeneratorCoM/12(dqj)
  qRef_ikin/1 -> Demux2/1
  Demux2/1 -> Terminator1/1
  Demux2/2 -> trajectoryGeneratorCoM/6(qj)

== system torqueBalancingJointControl/Define initial values/Inverse kinematics Solver/ikin visualizer ==
  Ikin_feetCorr : Inport
  Ikin_CoMCorr : Inport  Port=2
  Ikin_PostCorr : Inport  Port=3
  CoM Desired Dynamics : Scope
      settings: YMin=-0.045  YMax=0.045
  "Desired Posture " : Scope
      settings: YMin=0.0042  YMax=0.0055  SaveName=ScopeData4
  Feet Desired Dynamics : Scope
      settings: YMin=-3.75e-15  YMax=1.5e-15
  wires:
  Ikin_CoMCorr/1 -> CoM Desired Dynamics/1
  Ikin_feetCorr/1 -> Feet Desired Dynamics/1
  Ikin_PostCorr/1 -> "Desired Posture "/1

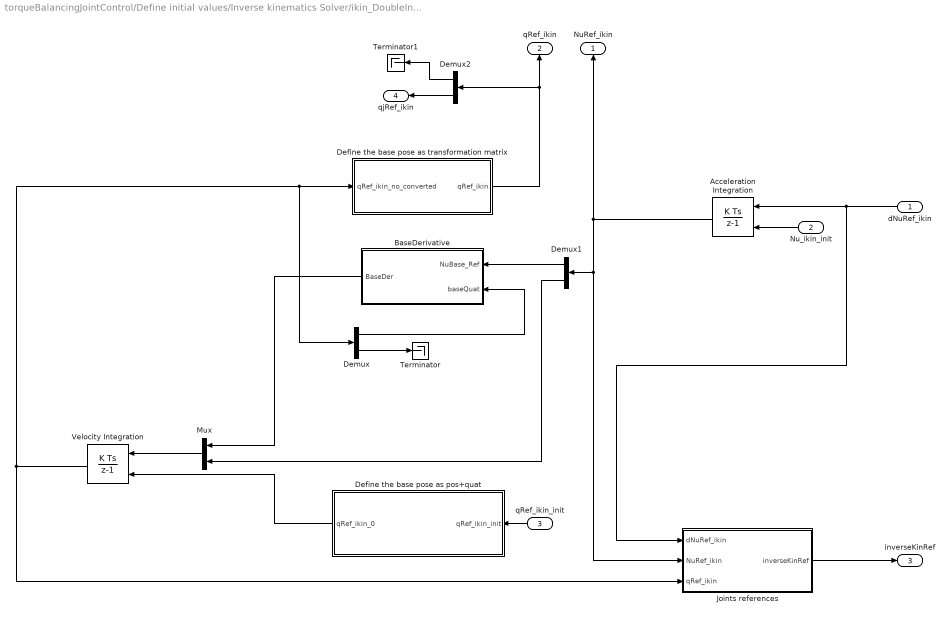
== system torqueBalancingJointControl/Define initial values/Inverse kinematics Solver/ikin_DoubleIntegrator ==
  dNuRef_ikin : Inport
  Nu_ikin_init : Inport  Port=2
  qRef_ikin_init : Inport  Port=3
  Acceleration Integration : DiscreteIntegrator  InitialConditionSource=external  SampleTime=CONFIG.Ts  ICPrevOutput=DiscIntNeverNeededParam  ICPrevScaledInput=DiscIntNeverNeededParam
  BaseDerivative : MATLAB Function  TreatAsAtomicUnit=on
  Define the base pose as pos+quat : MATLAB Function  TreatAsAtomicUnit=on
  Define the base pose as transformation matrix : MATLAB Function  TreatAsAtomicUnit=on
  Demux : Demux  Outputs=[7;ROBOT_DOF]
  Demux1 : Demux  Outputs=[6;ROBOT_DOF]
  Demux2 : Demux  Outputs=[16,ROBOT_DOF]
  Joints references : MATLAB Function  TreatAsAtomicUnit=on
  Mux : Mux  Inputs=2
  Terminator : Terminator
  Terminator1 : Terminator
  Velocity Integration : DiscreteIntegrator  InitialConditionSource=external  SampleTime=CONFIG.Ts  ICPrevOutput=DiscIntNeverNeededParam  ICPrevScaledInput=DiscIntNeverNeededParam
  NuRef_ikin : Outport
  qRef_ikin : Outport  Port=2
  inverseKinRef : Outport  Port=3
  qjRef_ikin : Outport  Port=4
  wires:
  Nu_ikin_init/1 -> Acceleration Integration/2
  qRef_ikin_init/1 -> Define the base pose as pos+quat/1(qRef_ikin_init)
  dNuRef_ikin/1 -> Joints references/1(dNuRef_ikin), Acceleration Integration/1
  Demux/2 -> Terminator/1
  Demux/1 -> BaseDerivative/2(baseQuat)
  Velocity Integration/1 -> Define the base pose as transformation matrix/1(qRef_ikin_no_converted), Demux/1, Joints references/3(qRef_ikin)
  Acceleration Integration/1 -> Joints references/2(NuRef_ikin), Demux1/1, NuRef_ikin/1
  Demux1/1 -> BaseDerivative/1(NuBase_Ref)
  BaseDerivative/1(BaseDer) -> Mux/1
  Demux1/2 -> Mux/2
  Mux/1 -> Velocity Integration/1
  Joints references/1(inverseKinRef) -> inverseKinRef/1
  Define the base pose as transformation matrix/1(qRef_ikin) -> Demux2/1, qRef_ikin/1
  Define the base pose as pos+quat/1(qRef_ikin_0) -> Velocity Integration/2
  Demux2/2 -> qjRef_ikin/1
  Demux2/1 -> Terminator1/1

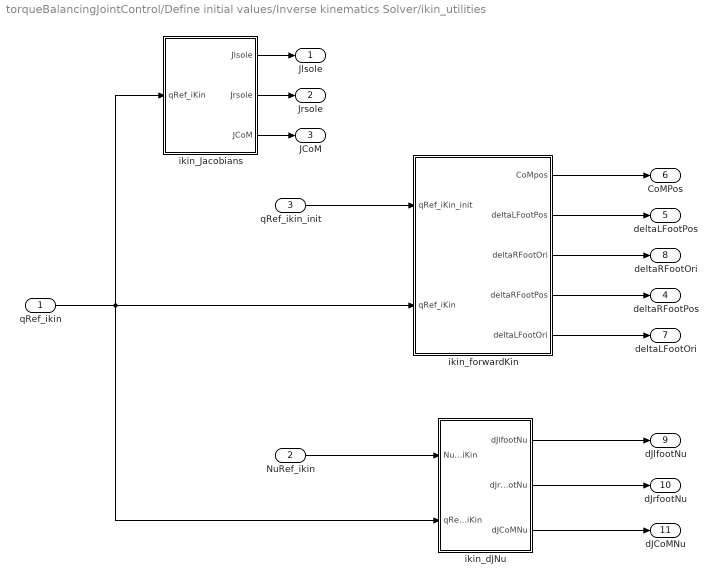
== system torqueBalancingJointControl/Define initial values/Inverse kinematics Solver/ikin_utilities ==
  qRef_ikin : Inport
  NuRef_ikin : Inport  Port=2
  qRef_ikin_init : Inport  Port=3
  ikin_Jacobians : Subsystem
  ikin_dJNu : Subsystem
  ikin_forwardKin : Subsystem
  Jlsole : Outport
  Jrsole : Outport  Port=2
  JCoM : Outport  Port=3
  deltaRFootPos : Outport  Port=4
  deltaLFootPos : Outport  Port=5
  CoMPos : Outport  Port=6
  deltaLFootOri : Outport  Port=7
  deltaRFootOri : Outport  Port=8
  dJlfootNu : Outport  Port=9
  dJrfootNu : Outport  Port=10
  dJCoMNu : Outport  Port=11
  wires:
  ikin_Jacobians/1(Jlsole) -> Jlsole/1
  ikin_Jacobians/3(JCoM) -> JCoM/1
  ikin_dJNu/3(dJCoMNu) -> dJCoMNu/1
  ikin_dJNu/1(dJlfootNu) -> dJlfootNu/1
  ikin_dJNu/2(dJrfootNu) -> dJrfootNu/1
  ikin_Jacobians/2(Jrsole) -> Jrsole/1
  qRef_ikin_init/1 -> ikin_forwardKin/1(qRef_iKin_init)
  qRef_ikin/1 -> ikin_Jacobians/1(qRef_iKin), ikin_dJNu/2(qRef_iKin), ikin_forwardKin/2(qRef_iKin)
  ikin_forwardKin/1(CoMpos) -> CoMPos/1
  ikin_forwardKin/2(deltaLFootPos) -> deltaLFootPos/1
  ikin_forwardKin/3(deltaRFootOri) -> deltaRFootOri/1
  ikin_forwardKin/4(deltaRFootPos) -> deltaRFootPos/1
  ikin_forwardKin/5(deltaLFootOri) -> deltaLFootOri/1
  NuRef_ikin/1 -> ikin_dJNu/1(NuRef_iKin)

== system torqueBalancingJointControl/Define initial values/References/q(0) ==
  qj : Inport
  "holder " : WBToolboxLibrary/Utilities/holder 
  l_sole_H_root_link : Subsystem
  w_H_b(0) : Outport
  qj(0) : Outport  Port=2
  wires:
  qj/1 -> "holder "/1
  "holder "/1 -> qj(0)/1, l_sole_H_root_link/1(qj)
  l_sole_H_root_link/1(l_sole_H_root_link) -> w_H_b(0)/1

== system torqueBalancingJointControl/Define initial values/References/xCom ==
  qj : Inport
  W_H_b : Inport  Port=2
  "CoM6D ->  CoMXYZ2" : Selector  NumberOfDimensions=2  InputPortWidth=7  IndexOptions=Index vector (dialog),Index vector (dialog)  Indices=[1 2 3],[4]  OutputSizes=1,1
  com : WBToolboxLibrary/wholeBodyModel/Kinematics/Forward Kinematics  frameName='com'  robotName=WBT_robotName  localName=WBT_modelName  wbiFile=WBT_wbiFilename  wbiList=WBT_wbiList
  xCom : Outport
  wires:
  qj/1 -> com/2
  "CoM6D ->  CoMXYZ2"/1 -> xCom/1
  com/1 -> "CoM6D ->  CoMXYZ2"/1
  W_H_b/1 -> com/1

== system torqueBalancingJointControl/Define initial values/Inverse kinematics Solver/ikin_utilities/ikin_Jacobians ==
  qRef_iKin : Inport
  Demux : Demux  Outputs=[16;ROBOT_DOF]
  Jacobian CoM : WBToolboxLibrary/wholeBodyModel/Jacobians/Jacobian  frameName='com'  robotName=WBT_robotName  localName=WBT_modelName  wbiFile=WBT_wbiFilename  wbiList=WBT_wbiList
  Jacobian l_foot : WBToolboxLibrary/wholeBodyModel/Jacobians/Jacobian  frameName='l_sole'  robotName=WBT_robotName  localName=WBT_modelName  wbiFile=WBT_wbiFilename  wbiList=WBT_wbiList
  Jacobian r_foot : WBToolboxLibrary/wholeBodyModel/Jacobians/Jacobian  frameName='r_sole'  robotName=WBT_robotName  localName=WBT_modelName  wbiFile=WBT_wbiFilename  wbiList=WBT_wbiList
  Reshape : Reshape  OutputDimensionality=Customize  OutputDimensions=[4,4]
  Jlsole : Outport
  Jrsole : Outport  Port=2
  JCoM : Outport  Port=3
  wires:
  qRef_iKin/1 -> Demux/1
  Demux/1 -> Reshape/1
  Reshape/1 -> Jacobian CoM/1, Jacobian r_foot/1, Jacobian l_foot/1
  Demux/2 -> Jacobian CoM/2, Jacobian r_foot/2, Jacobian l_foot/2
  Jacobian l_foot/1 -> Jlsole/1
  Jacobian r_foot/1 -> Jrsole/1
  Jacobian CoM/1 -> JCoM/1

== system torqueBalancingJointControl/Define initial values/Inverse kinematics Solver/ikin_utilities/ikin_dJNu ==
  NuRef_iKin : Inport
  qRef_iKin : Inport  Port=2
  Demux : Demux  Outputs=[16;ROBOT_DOF]
  Demux1 : Demux  Outputs=[6;ROBOT_DOF]
  DotJ Nu CoM : WBToolboxLibrary/wholeBodyModel/Jacobians/DotJ Nu  frameName='com'  robotName=WBT_robotName  localName=WBT_modelName  wbiFile=WBT_wbiFilename  wbiList=WBT_wbiList
  DotJ Nu Left foot : WBToolboxLibrary/wholeBodyModel/Jacobians/DotJ Nu  frameName='l_sole'  robotName=WBT_robotName  localName=WBT_modelName  wbiFile=WBT_wbiFilename  wbiList=WBT_wbiList
  DotJ Nu Right foot : WBToolboxLibrary/wholeBodyModel/Jacobians/DotJ Nu  frameName='r_sole'  robotName=WBT_robotName  localName=WBT_modelName  wbiFile=WBT_wbiFilename  wbiList=WBT_wbiList
  Reshape5 : Reshape  OutputDimensionality=Customize  OutputDimensions=[4,4]
  dJlfootNu : Outport
  dJrfootNu : Outport  Port=2
  dJCoMNu : Outport  Port=3
  wires:
  Demux1/1 -> DotJ Nu Right foot/3, DotJ Nu Left foot/3, DotJ Nu CoM/3
  Demux/1 -> Reshape5/1
  Reshape5/1 -> DotJ Nu CoM/1, DotJ Nu Right foot/1, DotJ Nu Left foot/1
  DotJ Nu CoM/1 -> dJCoMNu/1
  DotJ Nu Right foot/1 -> dJrfootNu/1
  DotJ Nu Left foot/1 -> dJlfootNu/1
  NuRef_iKin/1 -> Demux1/1
  qRef_iKin/1 -> Demux/1
  Demux/2 -> DotJ Nu Right foot/2, DotJ Nu Left foot/2, DotJ Nu CoM/2
  Demux1/2 -> DotJ Nu Right foot/4, DotJ Nu Left foot/4, DotJ Nu CoM/4

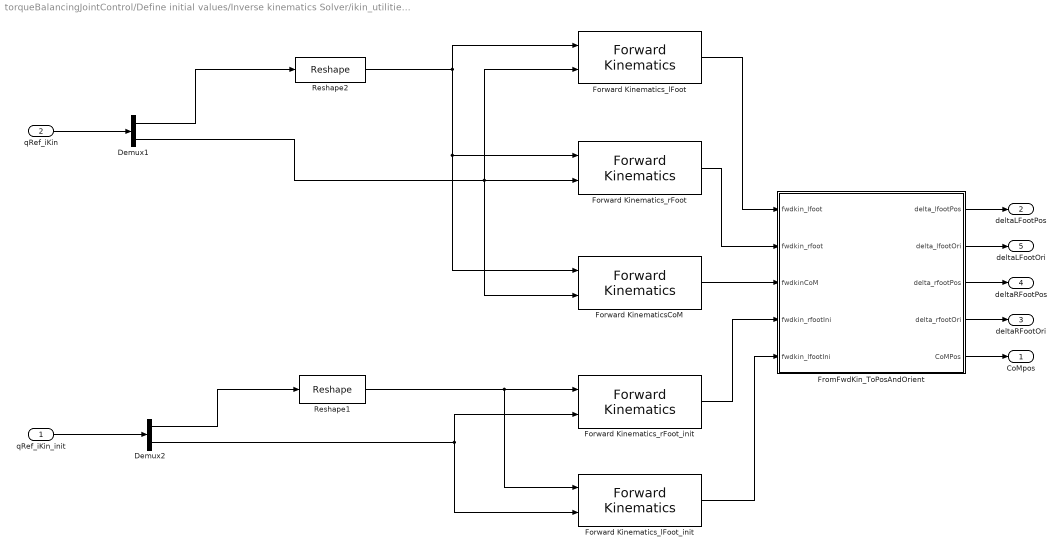
== system torqueBalancingJointControl/Define initial values/Inverse kinematics Solver/ikin_utilities/ikin_forwardKin ==
  qRef_iKin_init : Inport
  qRef_iKin : Inport  Port=2
  Demux1 : Demux  Outputs=[16;ROBOT_DOF]
  Demux2 : Demux  Outputs=[16;ROBOT_DOF]
  Forward KinematicsCoM : WBToolboxLibrary/wholeBodyModel/Kinematics/Forward Kinematics  frameName='com'  robotName=WBT_robotName  localName=WBT_modelName  wbiFile=WBT_wbiFilename  wbiList=WBT_wbiList
  Forward Kinematics_lFoot : WBToolboxLibrary/wholeBodyModel/Kinematics/Forward Kinematics  frameName='l_sole'  robotName=WBT_robotName  localName=WBT_modelName  wbiFile=WBT_wbiFilename  wbiList=WBT_wbiList
  Forward Kinematics_lFoot_init : WBToolboxLibrary/wholeBodyModel/Kinematics/Forward Kinematics  frameName='l_sole'  robotName=WBT_robotName  localName=WBT_modelName  wbiFile=WBT_wbiFilename  wbiList=WBT_wbiList
  Forward Kinematics_rFoot : WBToolboxLibrary/wholeBodyModel/Kinematics/Forward Kinematics  frameName='r_sole'  robotName=WBT_robotName  localName=WBT_modelName  wbiFile=WBT_wbiFilename  wbiList=WBT_wbiList
  Forward Kinematics_rFoot_init : WBToolboxLibrary/wholeBodyModel/Kinematics/Forward Kinematics  frameName='r_sole'  robotName=WBT_robotName  localName=WBT_modelName  wbiFile=WBT_wbiFilename  wbiList=WBT_wbiList
  FromFwdKin_ToPosAndOrient : MATLAB Function  TreatAsAtomicUnit=on
  Reshape1 : Reshape  OutputDimensionality=Customize  OutputDimensions=[4,4]
  Reshape2 : Reshape  OutputDimensionality=Customize  OutputDimensions=[4,4]
  CoMpos : Outport
  deltaLFootPos : Outport  Port=2
  deltaRFootOri : Outport  Port=3
  deltaRFootPos : Outport  Port=4
  deltaLFootOri : Outport  Port=5
  wires:
  qRef_iKin_init/1 -> Demux2/1
  Demux2/1 -> Reshape1/1
  qRef_iKin/1 -> Demux1/1
  Demux1/1 -> Reshape2/1
  Reshape2/1 -> Forward KinematicsCoM/1, Forward Kinematics_rFoot/1, Forward Kinematics_lFoot/1
  Reshape1/1 -> Forward Kinematics_lFoot_init/1, Forward Kinematics_rFoot_init/1
  Demux2/2 -> Forward Kinematics_lFoot_init/2, Forward Kinematics_rFoot_init/2
  Demux1/2 -> Forward KinematicsCoM/2, Forward Kinematics_lFoot/2, Forward Kinematics_rFoot/2
  Forward Kinematics_lFoot/1 -> FromFwdKin_ToPosAndOrient/1(fwdkin_lfoot)
  Forward Kinematics_rFoot/1 -> FromFwdKin_ToPosAndOrient/2(fwdkin_rfoot)
  Forward KinematicsCoM/1 -> FromFwdKin_ToPosAndOrient/3(fwdkinCoM)
  Forward Kinematics_rFoot_init/1 -> FromFwdKin_ToPosAndOrient/4(fwdkin_rfootIni)
  Forward Kinematics_lFoot_init/1 -> FromFwdKin_ToPosAndOrient/5(fwdkin_lfootIni)
  FromFwdKin_ToPosAndOrient/5(CoMPos) -> CoMpos/1
  FromFwdKin_ToPosAndOrient/1(delta_lfootPos) -> deltaLFootPos/1
  FromFwdKin_ToPosAndOrient/2(delta_lfootOri) -> deltaLFootOri/1
  FromFwdKin_ToPosAndOrient/3(delta_rfootPos) -> deltaRFootPos/1
  FromFwdKin_ToPosAndOrient/4(delta_rfootOri) -> deltaRFootOri/1

== system torqueBalancingJointControl/Define initial values/References/q(0)/l_sole_H_root_link ==
  qj : Inport
  Constant5 : Constant  Value=eye(4)
  Constant6 : Constant  Value=eye(4)
  Inv\* : Product  Inputs=/*  Multiplication=Matrix(*)
  l_sole : WBToolboxLibrary/wholeBodyModel/Kinematics/Forward Kinematics  frameName='l_sole'  robotName=WBT_robotName  localName=WBT_modelName  wbiFile=WBT_wbiFilename  wbiList=WBT_wbiList
  root_link : WBToolboxLibrary/wholeBodyModel/Kinematics/Forward Kinematics  frameName='root_link'  robotName=WBT_robotName  localName=WBT_modelName  wbiFile=WBT_wbiFilename  wbiList=WBT_wbiList
  l_sole_H_root_link : Outport
  wires:
  Constant5/1 -> l_sole/1
  Inv\*/1 -> l_sole_H_root_link/1  "l_sole_H_root_link"
  l_sole/1 -> Inv\*/1
  Constant6/1 -> root_link/1
  qj/1 -> l_sole/2, root_link/2
  root_link/1 -> Inv\*/2

== matlab function Define initial values/Inverse kinematics Solver/ikin_utilities/ikin_forwardKin/FromFwdKin_ToPosAndOrient ==
  data: fwdkin_lfoot input double; fwdkin_rfoot input double; fwdkinCoM input double; fwdkin_rfootIni input double; delta_lfootPos output double; fwdkin_lfootIni input double; delta_lfootOri output double; delta_rfootPos output double; delta_rfootOri output double; CoMPos output double
function [delta_lfootPos,delta_lfootOri,delta_rfootPos,delta_rfootOri,CoMPos] = fromFdwKinToPosOri(fwdkin_lfoot,fwdkin_rfoot,fwdkinCoM,fwdkin_rfootIni,...
                                                                                                   fwdkin_lfootIni)

[delta_lfootPos,delta_lfootOri,delta_rfootPos,delta_rfootOri,CoMPos] = FromFwdKinToPosAndOri(fwdkinCoM,fwdkin_lfoot,fwdkin_lfootIni,...
                                                                                             fwdkin_rfoot,fwdkin_rfootIni);
                                                                                         
end

== matlab function Define initial values/References/CoM Ref ==
  data: xCoM_ini input double; xCoMDes output double; t input double; referenceParams parameter double
function xCoMDes = genCoMRef(xCoM_ini,t,referenceParams)

desired_x_dx_ddx_CoM   = generateCoMTrajectory(xCoM_ini, t, referenceParams);
xCoMDes                = desired_x_dx_ddx_CoM(:,1);

end

== matlab function Define initial values/nu/genBaseVelocity ==
  data: JcLeftFoot input double; JcRightFoot input double; Constraints input double; Nu_base output double; dq input double; reg parameter double
function Nu_base = genBaseVel(JcLeftFoot,JcRightFoot,Constraints,dq,reg)

Nu_base = generateBaseVelocities(JcLeftFoot,JcRightFoot,Constraints,dq,reg);

end

== matlab function Define initial values/Inverse kinematics Solver/ikin_DoubleIntegrator/Define the base pose as transformation matrix ==
  data: qRef_ikin_no_converted input double; qRef_ikin output double
function qRef_ikin = baseToTransMatr(qRef_ikin_no_converted)

qRef_ikin = BasePoseToTransMatrix(qRef_ikin_no_converted);

end

== matlab function Define initial values/Inverse kinematics Solver/ikin_DoubleIntegrator/BaseDerivative ==
  data: NuBase_Ref input double; BaseDer output double; baseQuat input double
function BaseDer   = BaseDeriv(NuBase_Ref, baseQuat)

BaseDer   = BaseDerivative(NuBase_Ref, baseQuat);

end

== matlab function controller_JointSpace/tau(f)  ==
  data: tau output double; constraints input double; ConstraintsMatrix input double; bVectorConstraints input double; qj input double; Nu input double; inverseKinRef input double; M input double; h input double; Jc input double; dJcNu input double; impedances input double; reg parameter double; gain parameter double; fc output double
function [tau,fc]  = controller(constraints,ConstraintsMatrix,bVectorConstraints,qj,...
                                Nu,inverseKinRef, M,h , Jc, dJcNu, impedances,reg,gain)

[tau,fc]  = JointController(constraints, M, h, Jc, dJcNu,impedances, gain.dampings, inverseKinRef, qj,Nu,reg);

end

== matlab function Define initial values/Inverse kinematics Solver/ikin_DoubleIntegrator/Define the base pose as pos+quat ==
  data: qRef_ikin_init input double; qRef_ikin_0 output double
function qRef_ikin_0 = ConvStateToQuat(qRef_ikin_init)

qRef_ikin_0 = convertStateToQuat(qRef_ikin_init);

end

== matlab function Define initial values/Inverse kinematics Solver/ikin_DoubleIntegrator/Joints references ==
  data: dNuRef_ikin input double; inverseKinRef output double; NuRef_ikin input double; qRef_ikin input double
function inverseKinRef = fcn(dNuRef_ikin, NuRef_ikin, qRef_ikin)

inverseKinRef = generateJointRef(dNuRef_ikin, NuRef_ikin, qRef_ikin);

end

== matlab function system dynamics/Jacobians/composingSmoothJacobians ==
  data: constraints input double; JL input double; JR input double; Jc output double; dJLNu input double; dJRNu input double; dJcNu output double
function [Jc, dJcNu] = composingSmoothJacobians(constraints,JL,JR, dJLNu,dJRNu)

[Jc, dJcNu] = compSmoothJacobians(constraints,JL,JR, dJLNu,dJRNu);
      
end

== matlab function system dynamics/Centroidal tranformation/fromFloating2Centroidal ==
  data: M input double; M_c output double; h input double; g input double; Jc input double; dJcNu input double; Nu input double; c_T_b input double; dT input double; h_c output double; Jc_c output double; dJcNu_c output double; Nu_c output double
function [M_c,h_c, Jc_c, dJcNu_c, Nu_c] = fromFloating2Centroidal(M, h, g, Jc, dJcNu, Nu, c_T_b, dT)

[M_c,C_cNu_c, g_c, Jc_c, dJcNu_c, Nu_c] = fromFloatingToCentroidalDynamics(M, h, g, Jc, dJcNu, Nu, c_T_b, dT);

 h_c = C_cNu_c + g_c;

end

== matlab function system dynamics/Centroidal tranformation/fromState2TandTD ==
  data: M input double; xcom input double; c_T_b output double; wHb input double; dxcom input double; dx_b input double; dT output double
function [c_T_b, dT] = centroidalTransformationT_TDot(M,xcom,wHb,dxcom,dx_b)

[c_T_b, dT] = centroidalTransformationT_TDot(xcom,wHb(1:3,4),dxcom,dx_b,M);

end

== matlab function Define initial values/Inverse kinematics Solver/trajectoryGeneratorCoM ==
  data: iKinFeetCorr input double; iKinComCorr input double; iKinPostCorr input double; J_lfoot input double; J_rfoot input double; J_com input double; dNuRef_ikin output double; dJcNu_lf input double; dJcNu_rf input double; dJ_comNu input double; constraints input double
function dNuRef_ikin   = ikin_AccelerationRef_generator(iKinFeetCorr, iKinComCorr, iKinPostCorr, J_lfoot, J_rfoot, J_com, dJcNu_lf,...
                                                       dJcNu_rf, dJ_comNu, constraints)

n_joints = size(J_com(:,7:end),2);

%% jacobians and jacobian derivatives
JFeet      = [constraints(1)*J_lfoot ; constraints(2)*J_rfoot];
JCoM       = J_com(1:3,:);
JPosture   = [zeros(n_joints,6),eye(n_joints)]; 

dJFeetNu   = [constraints(1)*dJcNu_lf; constraints(2)*dJcNu_rf];
dJCoMNu    = dJ_comNu(1:3);

%% state acceleration reference calculation
dNuRef_ikin = Ikin_AccelerationRef_generator(JFeet, JCoM, JPosture, dJFeetNu, dJCoMNu, iKinFeetCorr, iKinComCorr, iKinPostCorr); 

end

== matlab function Define initial values/Inverse kinematics Solver/Generate ikin Errors/trajectoryGeneratorCoM ==
  data: lFootPos input double; rFootPos input double; rFootOri input double; lFootOri input double; xCoM input double; qj input double; CoMRefsDes input double; posturesDes input double; lFootVel input double; rFootVel input double; dxCoM input double; dqj input double; iKinFeetCorr output double; iKinComCorr output double; iKinPostCorr output double; gain parameter double
function [iKinFeetCorr,iKinComCorr,iKinPostCorr]  = ikin_PosAndOriErrors(lFootPos,rFootPos,rFootOri,lFootOri,xCoM,qj, CoMRefsDes,posturesDes,lFootVel,...
                                                                         rFootVel,dxCoM,dqj,gain)

[iKinFeetCorr,iKinComCorr,iKinPostCorr]  = ikin_PosAndOrientErrors(lFootPos,rFootPos,rFootOri,lFootOri,xCoM,qj, CoMRefsDes,posturesDes,...
                                                                            lFootVel,rFootVel,dxCoM,dqj,gain);

end
